simulink model "US7259704"  (R2017a)
settings: Solver=FixedStepAuto  StartTime=0.0  StopTime=0.1  RelTol=1e-3  EnableMultiTasking=on
libraries: dspmlti4 x8, dsparch4 x1
settings Model: Creator=bhannigan  LastModifiedBy=bhannigan
settings OptimizationCC: LifeSpan=inf
settings DebuggingCC: SFUnexpectedBacktrackingDiag=warning  SFNoUnconditionalDefaultTransitionDiag=warning  SFExecutionAtInitializationDiag=none
settings GRTTargetCC: TargetLangStandard=C89/C90 (ANSI)  GeneratePreprocessorConditionals=Disable all
settings ConfigComp: CovMetricSettings=dw  CovHtmlReporting=on  CovSaveCumulativeToWorkspaceVar=on  CovSaveSingleToWorkspaceVar=on  CovExternalEMLEnable=off

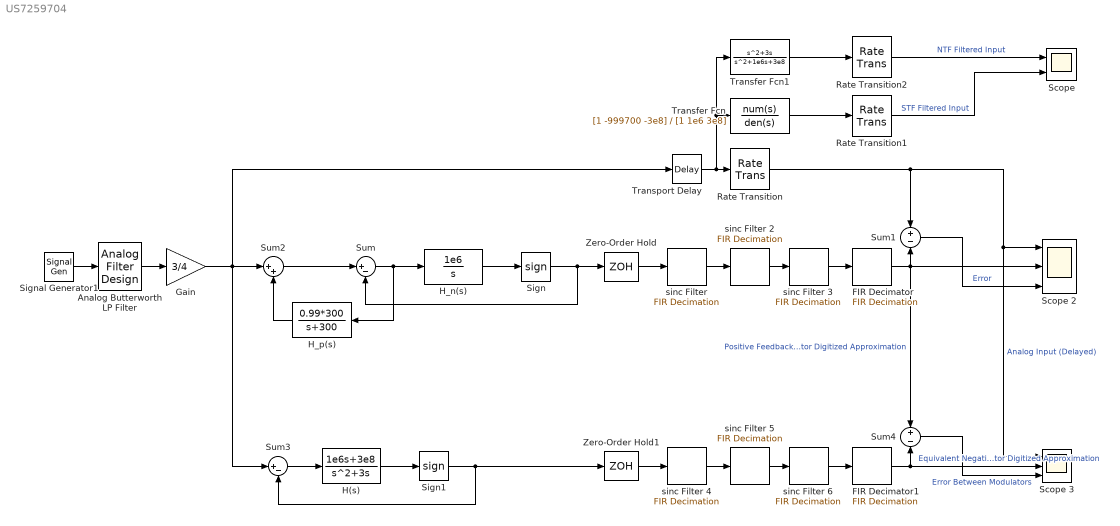
== system US7259704 ==
  Analog Butterworth LP Filter : dsparch4/Analog Filter Design  method=Butterworth  filttype=Lowpass  N=5  Wlo=2*pi*400  Whi=80  Rp=2  Rs=40
  FIR Decimator : dspmlti4/FIR Decimation  FilterSource=Dialog parameters  h=fir1(63, 0.25)  D=4  filtStruct=Direct form  FilterObject=Hm_firdecim  framing=Allow multirate processing  inputOffset=0  outputBufInitCond=0  roundingMode=Floor  overflowMode=off  firstCoeffDataTypeStr=Inherit: Same word length as input  firstCoeffMin=[]  firstCoeffMax=[]  firstCoeffLastDataTypeStr=Inherit: Same word length as input  accumDataTypeStr=Inherit: Same as product output  accumLastDataTypeStr=Inherit: Same as product output  outputMin=[]  outputMax=[]
  FIR Decimator1 : dspmlti4/FIR Decimation  FilterSource=Dialog parameters  h=fir1(63, 0.25)  D=4  filtStruct=Direct form  FilterObject=Hm_firdecim  framing=Allow multirate processing  inputOffset=0  outputBufInitCond=0  roundingMode=Floor  overflowMode=off  firstCoeffDataTypeStr=Inherit: Same word length as input  firstCoeffMin=[]  firstCoeffMax=[]  firstCoeffLastDataTypeStr=Inherit: Same word length as input  accumDataTypeStr=Inherit: Same as product output  accumLastDataTypeStr=Inherit: Same as product output  outputMin=[]  outputMax=[]
  Gain : Gain  Gain=3/4  SaturateOnIntegerOverflow=on  OutDataTypeStr=Inherit: Same as input  ParamDataTypeStr=Inherit: Same as input
  H(s) : TransferFcn  Numerator=[1e6 3e8]  Denominator=[1 3 0]
  H_n(s) : TransferFcn  Numerator=1e6  Denominator=[1 0]
  H_p(s) : TransferFcn  Numerator=0.99*300  Denominator=[1 300]
  Rate Transition : RateTransition
  Rate Transition1 : RateTransition
  Rate Transition2 : RateTransition
  Scope : Scope  NumInputPorts=2
  Scope 2 : Scope  NumInputPorts=3
  Scope 3 : Scope  NumInputPorts=3
  Sign : Signum
  Sign1 : Signum
  Signal Generator1 : SignalGenerator  WaveForm=square  Frequency=80
  Sum : Sum  Inputs=|+-
  Sum1 : Sum  Inputs=+-  SaturateOnIntegerOverflow=on  InputSameDT=on  OutDataTypeStr=Inherit: Same as first input
  Sum2 : Sum  Inputs=|++
  Sum3 : Sum  Inputs=|+-
  Sum4 : Sum  Inputs=+-  SaturateOnIntegerOverflow=on  InputSameDT=on  OutDataTypeStr=Inherit: Same as first input
  Transfer Fcn : TransferFcn  Numerator=[1 -999700 -3e8]  Denominator=[1 1e6 3e8]
  Transfer Fcn1 : TransferFcn  Numerator=[1 3 0]  Denominator=[1 1e6 3e8]
  Transport Delay : TransportDelay  DelayTime=736/512000
  Zero-Order Hold : ZeroOrderHold  SampleTime=1/512000
  Zero-Order Hold1 : ZeroOrderHold  SampleTime=1/512000
  sinc Filter : dspmlti4/FIR Decimation  FilterSource=Dialog parameters  h=1/64*ones(1, 64)  D=2  filtStruct=Direct form  FilterObject=Hm_firdecim  framing=Allow multirate processing  inputOffset=0  outputBufInitCond=0  roundingMode=Floor  overflowMode=off  firstCoeffDataTypeStr=Inherit: Same word length as input  firstCoeffMin=[]  firstCoeffMax=[]  firstCoeffLastDataTypeStr=Inherit: Same word length as input  accumDataTypeStr=Inherit: Same as product output  accumLastDataTypeStr=Inherit: Same as product output  outputMin=[]  outputMax=[]
  sinc Filter 2 : dspmlti4/FIR Decimation  FilterSource=Dialog parameters  h=1/64*ones(1, 64)  D=2  filtStruct=Direct form  FilterObject=Hm_firdecim  framing=Allow multirate processing  inputOffset=0  outputBufInitCond=0  roundingMode=Floor  overflowMode=off  firstCoeffDataTypeStr=Inherit: Same word length as input  firstCoeffMin=[]  firstCoeffMax=[]  firstCoeffLastDataTypeStr=Inherit: Same word length as input  accumDataTypeStr=Inherit: Same as product output  accumLastDataTypeStr=Inherit: Same as product output  outputMin=[]  outputMax=[]
  sinc Filter 3 : dspmlti4/FIR Decimation  FilterSource=Dialog parameters  h=1/64*ones(1, 64)  D=4  filtStruct=Direct form  FilterObject=Hm_firdecim  framing=Allow multirate processing  inputOffset=0  outputBufInitCond=0  roundingMode=Floor  overflowMode=off  firstCoeffDataTypeStr=Inherit: Same word length as input  firstCoeffMin=[]  firstCoeffMax=[]  firstCoeffLastDataTypeStr=Inherit: Same word length as input  accumDataTypeStr=Inherit: Same as product output  accumLastDataTypeStr=Inherit: Same as product output  outputMin=[]  outputMax=[]
  sinc Filter 4 : dspmlti4/FIR Decimation  FilterSource=Dialog parameters  h=1/64*ones(1, 64)  D=2  filtStruct=Direct form  FilterObject=Hm_firdecim  framing=Allow multirate processing  inputOffset=0  outputBufInitCond=0  roundingMode=Floor  overflowMode=off  firstCoeffDataTypeStr=Inherit: Same word length as input  firstCoeffMin=[]  firstCoeffMax=[]  firstCoeffLastDataTypeStr=Inherit: Same word length as input  accumDataTypeStr=Inherit: Same as product output  accumLastDataTypeStr=Inherit: Same as product output  outputMin=[]  outputMax=[]
  sinc Filter 5 : dspmlti4/FIR Decimation  FilterSource=Dialog parameters  h=1/64*ones(1, 64)  D=2  filtStruct=Direct form  FilterObject=Hm_firdecim  framing=Allow multirate processing  inputOffset=0  outputBufInitCond=0  roundingMode=Floor  overflowMode=off  firstCoeffDataTypeStr=Inherit: Same word length as input  firstCoeffMin=[]  firstCoeffMax=[]  firstCoeffLastDataTypeStr=Inherit: Same word length as input  accumDataTypeStr=Inherit: Same as product output  accumLastDataTypeStr=Inherit: Same as product output  outputMin=[]  outputMax=[]
  sinc Filter 6 : dspmlti4/FIR Decimation  FilterSource=Dialog parameters  h=1/64*ones(1, 64)  D=4  filtStruct=Direct form  FilterObject=Hm_firdecim  framing=Allow multirate processing  inputOffset=0  outputBufInitCond=0  roundingMode=Floor  overflowMode=off  firstCoeffDataTypeStr=Inherit: Same word length as input  firstCoeffMin=[]  firstCoeffMax=[]  firstCoeffLastDataTypeStr=Inherit: Same word length as input  accumDataTypeStr=Inherit: Same as product output  accumLastDataTypeStr=Inherit: Same as product output  outputMin=[]  outputMax=[]
  wires:
  Analog Butterworth LP Filter/1 -> Gain/1
  Signal Generator1/1 -> Analog Butterworth LP Filter/1
  Gain/1 -> Sum3/1, Sum2/1, Transport Delay/1
  Transport Delay/1 -> Transfer Fcn1/1, Transfer Fcn/1, Rate Transition/1
  Sign/1 -> Zero-Order Hold/1, Sum/2
  Rate Transition/1 -> Sum1/1, Scope 3/1, Scope 2/1  "Analog Input (Delayed)"
  sinc Filter 2/1 -> sinc Filter 3/1
  sinc Filter/1 -> sinc Filter 2/1
  sinc Filter 3/1 -> FIR Decimator/1
  FIR Decimator/1 -> Sum4/1, Sum1/2, Scope 2/2  "Positive Feedback Modulator Digitized Approximation"
  H_n(s)/1 -> Sign/1
  Sum/1 -> H_n(s)/1, H_p(s)/1
  H_p(s)/1 -> Sum2/2
  Sum2/1 -> Sum/1
  Zero-Order Hold/1 -> sinc Filter/1
  Transfer Fcn/1 -> Rate Transition1/1
  Transfer Fcn1/1 -> Rate Transition2/1
  Sign1/1 -> Zero-Order Hold1/1, Sum3/2
  sinc Filter 5/1 -> sinc Filter 6/1
  sinc Filter 4/1 -> sinc Filter 5/1
  sinc Filter 6/1 -> FIR Decimator1/1
  Zero-Order Hold1/1 -> sinc Filter 4/1
  H(s)/1 -> Sign1/1
  Sum3/1 -> H(s)/1
  FIR Decimator1/1 -> Sum4/2, Scope 3/2  "Equivalent Negative Feedback Modulator Digitized Approximation"
  Rate Transition2/1 -> Scope/1  "NTF Filtered Input"
  Rate Transition1/1 -> Scope/2  "STF Filtered Input"
  Sum1/1 -> Scope 2/3  "Error"
  Sum4/1 -> Scope 3/3  "Error Between Modulators"
